simulink model "PruebaMPC"  (R2021b)
settings: Solver=VariableStepDiscrete  StartTime=0.0  StopTime=Tsim  MaxStep=Ts  RelTol=1e-3
InitFcn:
  | init_fcn
values from neighbouring files (symbols this model uses):
  ss2 = c2d(ss2c, T_pred, 'tustin')    [init_fcn.m]
  T_ext = 15    [init_fcn.m]
  T_pred = Ts    (= 0.0005)    [init_fcn.m]
undefined symbols (not defined in the file or in its folder): F, K, Kobs, M, N, N2, Q, Temp_ref, Tsim, U0, X0
settings Model: Creator=martalopez  LastModifiedBy=martalopez
settings DataIOCC: ReturnWorkspaceOutputs=off

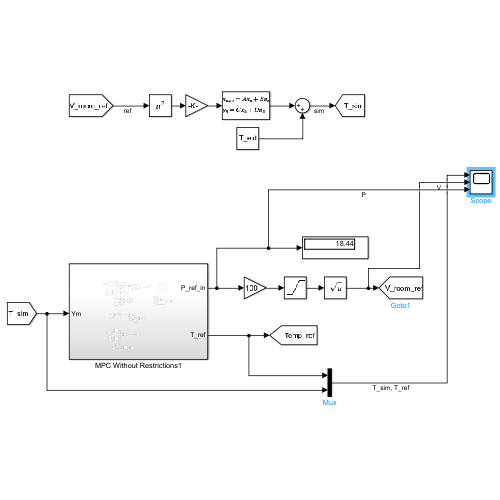
[thumbnail: Simulink's stored preview of the top-level diagram]
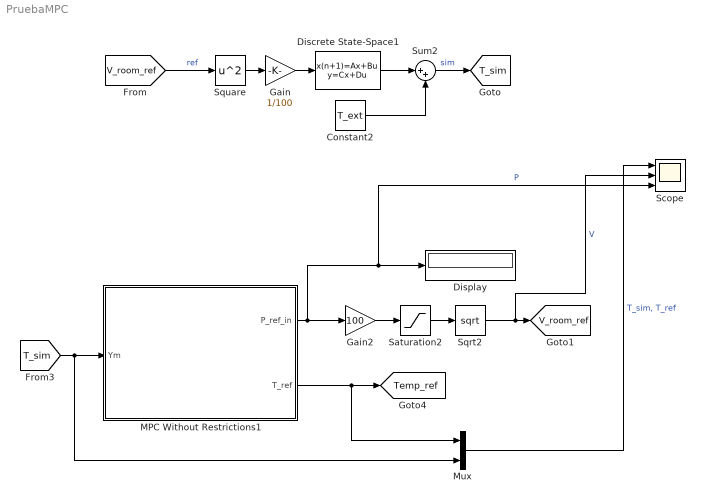
== system PruebaMPC ==
  Constant2 : Constant  Value=T_ext
  Discrete State-Space1 : DiscreteStateSpace  A=ss2.A  B=ss2.B  C=ss2.C  D=ss2.D  SampleTime=T_pred
  Display : Display
  Gain : Gain  Gain=1/100
  Gain2 : Gain  Gain=100
  MPC Without Restrictions1 : Subsystem
  Mux : Mux  Inputs=2
  Saturation2 : Saturate  UpperLimit=inf  LowerLimit=0
  Scope : Scope  NumInputPorts=3
  Sqrt2 : Sqrt  SaturateOnIntegerOverflow=on
  Square : Math  Operator=square  SaturateOnIntegerOverflow=on
  Sum2 : Sum  Inputs=|++
  tag scope: T_sim=global, Temp_ref=global, V_room_ref=global
  wires:
  [V_room_ref] -> Square/1  "ref"
  Discrete State-Space1/1 -> Sum2/1
  Gain/1 -> Discrete State-Space1/1
  Constant2/1 -> Sum2/2
  Square/1 -> Gain/1
  Sum2/1 -> [T_sim]  "sim"
  Sqrt2/1 -> Scope/2, [V_room_ref]  "V"
  [T_sim] -> Mux/2, MPC Without Restrictions1/1(Ym)
  MPC Without Restrictions1/2(T_ref) -> Mux/1, [Temp_ref]
  Saturation2/1 -> Sqrt2/1
  Gain2/1 -> Saturation2/1
  MPC Without Restrictions1/1(P_ref_in) -> Gain2/1, Scope/3, Display/1  "P"
  Mux/1 -> Scope/1  "T_sim, T_ref"

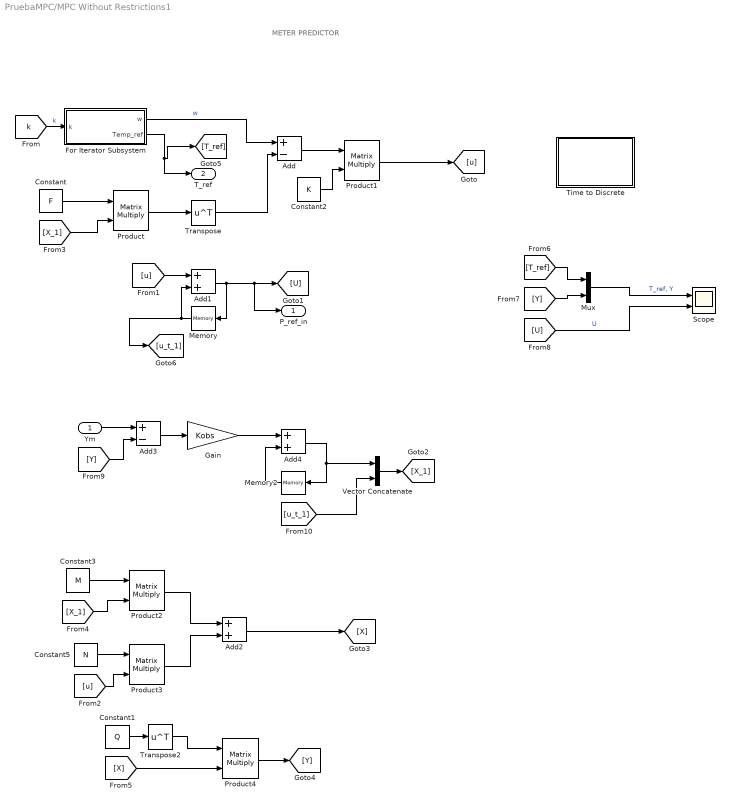
== system PruebaMPC/MPC Without Restrictions1 ==
  note: METER PREDICTOR
  Ym : Inport
  Add : Sum  Inputs=+-
  Add1 : Sum
  Add2 : Sum
  Add3 : Sum  Inputs=+-
  Add4 : Sum
  Constant : Constant  Value=F
  Constant1 : Constant  Value=Q
  Constant2 : Constant  Value=K
  Constant3 : Constant  Value=M
  Constant5 : Constant  Value=N
  For Iterator Subsystem : Subsystem  TreatAsAtomicUnit=on
  Gain : Gain  Gain=Kobs
  Memory : Memory  InitialCondition=U0
  Memory2 : Memory  InitialCondition=X0
  Mux : Mux  Inputs=2
  Product{,1..4} (5 alike) : Product  Multiplication=Matrix(*)
  Scope : Scope  NumInputPorts=2
  Time to Discrete : Subsystem
  Transpose : Math  Operator=transpose  SaturateOnIntegerOverflow=on
  Transpose2 : Math  Operator=transpose  SaturateOnIntegerOverflow=on
  Vector Concatenate : Concatenate
  P_ref_in : Outport
  T_ref : Outport  Port=2
  wires:
  Transpose2/1 -> Product4/1
  [u] -> Product3/2
  [u] -> Add1/1
  Memory/1 -> Add1/2, [u_t_1]
  Add2/1 -> [X]
  Transpose/1 -> Add/2
  Product/1 -> Transpose/1
  Constant5/1 -> Product3/1
  Product3/1 -> Add2/2
  Product2/1 -> Add2/1
  [X_1] -> Product2/2
  [X_1] -> Product/2
  Constant1/1 -> Transpose2/1
  Add/1 -> Product1/1
  For Iterator Subsystem/2(Temp_ref) -> [T_ref], T_ref/1
  Constant2/1 -> Product1/2
  [U] -> Scope/2  "U"
  [k] -> For Iterator Subsystem/1(k)  "k"
  For Iterator Subsystem/1(w) -> Add/1  "w"
  Constant3/1 -> Product2/1
  [T_ref] -> Mux/1
  [Y] -> Mux/2
  Constant/1 -> Product/1
  Mux/1 -> Scope/1  "T_ref, Y"
  Product4/1 -> [Y]
  Product1/1 -> [u]
  [X] -> Product4/2
  Add1/1 -> P_ref_in/1, [U], Memory/1
  Ym/1 -> Add3/1
  [Y] -> Add3/2
  Add3/1 -> Gain/1
  Gain/1 -> Add4/1
  Add4/1 -> Vector Concatenate/1, Memory2/1
  Memory2/1 -> Add4/2
  [u_t_1] -> Vector Concatenate/2
  Vector Concatenate/1 -> [X_1]

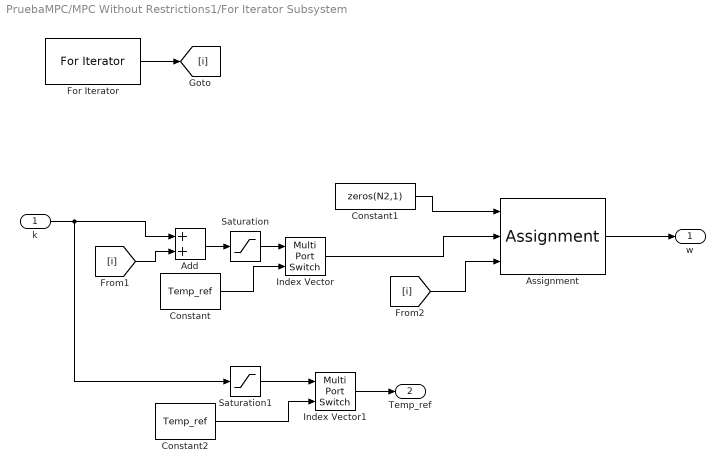
== system PruebaMPC/MPC Without Restrictions1/For Iterator Subsystem ==
  k : Inport
  Add : Sum
  Assignment : Assignment  IndexMode=Zero-based  DiagnosticForDimensions=Warning  IndexOptions=Index vector (port)  Indices=1  OutputSizes=1
  Constant : Constant  Value=Temp_ref
  Constant1 : Constant  Value=zeros(N2,1)
  Constant2 : Constant  Value=Temp_ref
  For Iterator : ForIterator  IterationLimit=N2  IndexMode=Zero-based
  Index Vector : MultiPortSwitch  DataPortOrder=Zero-based contiguous  Inputs=1  zeroidx=on
  Index Vector1 : MultiPortSwitch  DataPortOrder=Zero-based contiguous  Inputs=1  zeroidx=on
  Saturation : Saturate  UpperLimit=(Tsim/T_pred)-1  LowerLimit=0
  Saturation1 : Saturate  UpperLimit=(Tsim/T_pred)-1  LowerLimit=0
  w : Outport
  Temp_ref : Outport  Port=2
  wires:
  Saturation/1 -> Index Vector/1
  Constant/1 -> Index Vector/2
  For Iterator/1 -> [i]
  Add/1 -> Saturation/1
  [i] -> Add/2
  k/1 -> Saturation1/1, Add/1
  Constant1/1 -> Assignment/1
  Index Vector/1 -> Assignment/2
  Assignment/1 -> w/1
  [i] -> Assignment/3
  Constant2/1 -> Index Vector1/2
  Index Vector1/1 -> Temp_ref/1
  Saturation1/1 -> Index Vector1/1

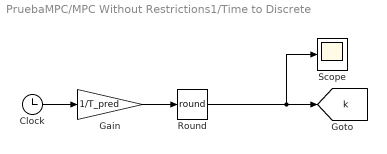
== system PruebaMPC/MPC Without Restrictions1/Time to Discrete ==
  Clock : Clock
  Gain : Gain  Gain=1/T_pred
  Round : Rounding  Operator=round
  Scope : Scope
  tag scope: k=global
  wires:
  Clock/1 -> Gain/1
  Gain/1 -> Round/1
  Round/1 -> [k], Scope/1
